simulink model "app_Main1msMgr"  (R2019b)
settings: Solver=FixedStepDiscrete  StartTime=0.0  StopTime=inf  FixedStep=0.001  RelTol=1e-3  EnableMultiTasking=on
PreLoadFcn:
  | try
  |    tapas_types('load');
  | catch
  |   disp('TAPAS WARNING: Tapas Types could not be loaded ...');
  | end
  | 
  | try
  |   app_types('load');
  | catch
  |   currdir =pwd;
  |   try
  |     cd('..\app_types\');
  |     app_types('load');
  |     cd(currdir);
  |   catch
  |     try
  |        cd('..\..\app_types\');
  |        app_types('load');
  |        cd(currdir);
  |     catch
  |        cd(currdir);
  |        disp('TAPAS WARNING: Application Types could not be loaded ...');
  |     end
  |   end
  |   try
  |       clear currdir;
  |   catch
  |      %Do nothing
  |   end
  | end
settings Model: Creator=kmansour  LastModifiedBy=depl_
settings DataIOCC: LimitDataPoints=on  SaveFormat=Array  ReturnWorkspaceOutputs=off
settings OptimizationCC: LifeSpan=1  EfficientTunableParamExpr=on
settings DebuggingCC: AllowSymbolicDim=off  SFUnexpectedBacktrackingDiag=warning  SFNoUnconditionalDefaultTransitionDiag=warning  SFExecutionAtInitializationDiag=none  ArithmeticOperatorsInVariantConditions=warning
settings HardwareCC: ProdBitPerPointer=32  ProdBitPerSizeT=32  ProdBitPerPtrDiffT=32  ProdLargestAtomicInteger=Long  ProdLargestAtomicFloat=Double  ProdEndianess=BigEndian  ProdWordSize=32  ProdHWDeviceType=Texas Instruments->TMS570 Cortex-R4
settings ModelReferenceCC: ModelReferenceNumInstancesAllowed=Single  PropagateSignalLabelsOutOfModel=off
settings SFSimCC: SimUseLocalCustomCode=off  MATLABDynamicMemAlloc=off  CustomCodeUndefinedFunction=UseInterfaceOnly
settings RTWCC: SystemTargetFile=ert.tlc  GenCodeOnly=on  TemplateMakefile=ert_default_tmf  GenerateReport=on  RTWUseLocalCustomCode=off  IncludeHyperlinkInReport=on  LaunchReport=on  GenerateTraceInfo=on  GenerateTraceReport=on  GenerateTraceReportSl=on  GenerateTraceReportSf=on  GenerateTraceReportEml=on
settings CodeAppCC: IgnoreCustomStorageClasses=off  MaxIdLength=63  StateflowObjectComments=on
settings ERTTargetCC: MultiwordLength=2048  GenerateSampleERTMain=on  GenerateASAP2=on  RTWCAPISignals=on  RTWCAPIParams=on  RTWCAPIStates=on  RTWCAPIRootIO=on  ERTSrcFileBannerTemplate=deMCD_code_template.cgt  ERTHdrFileBannerTemplate=deMCD_code_template.cgt  ERTDataSrcFileTemplate=deMCD_code_template.cgt  ERTDataHdrFileTemplate=deMCD_code_template.cgt  ERTCustomFileTemplate=example_file_process.tlc  ConvertIfToSwitch=off  SuppressUnreachableDefaultCases=off
settings ConfigComp: CovMetricSettings=dw  CovHtmlReporting=on  CovSaveCumulativeToWorkspaceVar=on  CovSaveSingleToWorkspaceVar=on  CovExternalEMLEnable=off

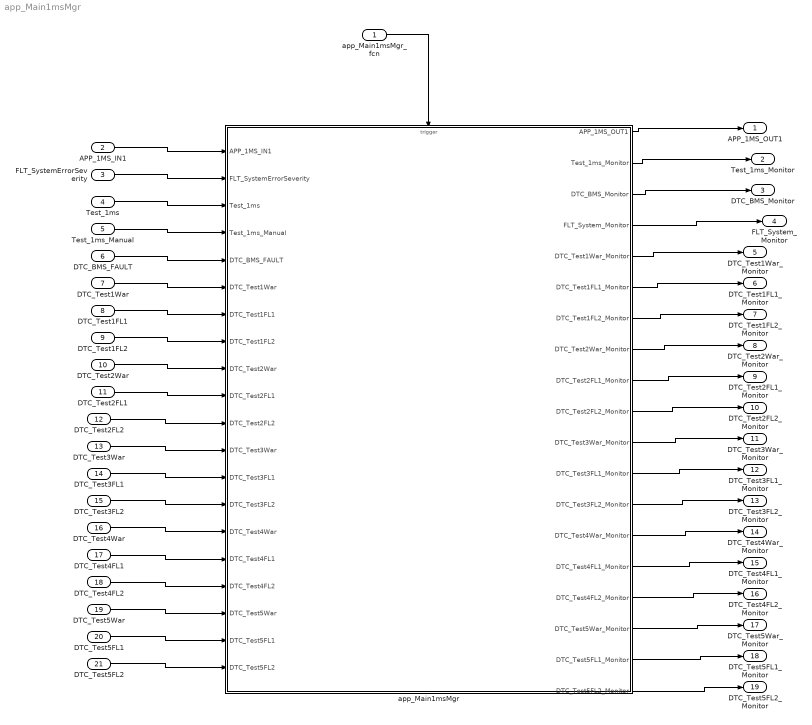
== system app_Main1msMgr ==
  app_Main1msMgr_fcn : Inport  SampleTime=1e-3  OutputFunctionCall=on
  APP_1MS_IN1 : Inport  Port=2
  FLT_SystemErrorSeverity : Inport  Port=3
  Test_1ms : Inport  Port=4
  Test_1ms_Manual : Inport  Port=5
  DTC_BMS_FAULT : Inport  Port=6
  DTC_Test1War : Inport  Port=7
  DTC_Test1FL1 : Inport  Port=8
  DTC_Test1FL2 : Inport  Port=9
  DTC_Test2War : Inport  Port=10
  DTC_Test2FL1 : Inport  Port=11
  DTC_Test2FL2 : Inport  Port=12
  DTC_Test3War : Inport  Port=13
  DTC_Test3FL1 : Inport  Port=14
  DTC_Test3FL2 : Inport  Port=15
  DTC_Test4War : Inport  Port=16
  DTC_Test4FL1 : Inport  Port=17
  DTC_Test4FL2 : Inport  Port=18
  DTC_Test5War : Inport  Port=19
  DTC_Test5FL1 : Inport  Port=20
  DTC_Test5FL2 : Inport  Port=21
  app_Main1msMgr : Subsystem
      mask Display: image(('Devise Logo.JPG'),'center');
  APP_1MS_OUT1 : Outport
  Test_1ms_Monitor : Outport  Port=2
  DTC_BMS_Monitor : Outport  Port=3
  FLT_System_Monitor : Outport  Port=4
  DTC_Test1War_Monitor : Outport  Port=5
  DTC_Test1FL1_Monitor : Outport  Port=6
  DTC_Test1FL2_Monitor : Outport  Port=7
  DTC_Test2War_Monitor : Outport  Port=8
  DTC_Test2FL1_Monitor : Outport  Port=9
  DTC_Test2FL2_Monitor : Outport  Port=10
  DTC_Test3War_Monitor : Outport  Port=11
  DTC_Test3FL1_Monitor : Outport  Port=12
  DTC_Test3FL2_Monitor : Outport  Port=13
  DTC_Test4War_Monitor : Outport  Port=14
  DTC_Test4FL1_Monitor : Outport  Port=15
  DTC_Test4FL2_Monitor : Outport  Port=16
  DTC_Test5War_Monitor : Outport  Port=17
  DTC_Test5FL1_Monitor : Outport  Port=18
  DTC_Test5FL2_Monitor : Outport  Port=19
  wires:
  app_Main1msMgr_fcn/1 -> app_Main1msMgr/Trigger
  APP_1MS_IN1/1 -> app_Main1msMgr/1(APP_1MS_IN1)
  app_Main1msMgr/1(APP_1MS_OUT1) -> APP_1MS_OUT1/1
  FLT_SystemErrorSeverity/1 -> app_Main1msMgr/2(FLT_SystemErrorSeverity)
  Test_1ms/1 -> app_Main1msMgr/3(Test_1ms)
  app_Main1msMgr/2(Test_1ms_Monitor) -> Test_1ms_Monitor/1
  Test_1ms_Manual/1 -> app_Main1msMgr/4(Test_1ms_Manual)
  app_Main1msMgr/3(DTC_BMS_Monitor) -> DTC_BMS_Monitor/1
  app_Main1msMgr/4(FLT_System_Monitor) -> FLT_System_Monitor/1
  DTC_BMS_FAULT/1 -> app_Main1msMgr/5(DTC_BMS_FAULT)
  DTC_Test1War/1 -> app_Main1msMgr/6(DTC_Test1War)
  DTC_Test1FL1/1 -> app_Main1msMgr/7(DTC_Test1FL1)
  DTC_Test1FL2/1 -> app_Main1msMgr/8(DTC_Test1FL2)
  DTC_Test2War/1 -> app_Main1msMgr/9(DTC_Test2War)
  DTC_Test2FL1/1 -> app_Main1msMgr/10(DTC_Test2FL1)
  DTC_Test2FL2/1 -> app_Main1msMgr/11(DTC_Test2FL2)
  DTC_Test3War/1 -> app_Main1msMgr/12(DTC_Test3War)
  DTC_Test3FL1/1 -> app_Main1msMgr/13(DTC_Test3FL1)
  DTC_Test3FL2/1 -> app_Main1msMgr/14(DTC_Test3FL2)
  DTC_Test4War/1 -> app_Main1msMgr/15(DTC_Test4War)
  DTC_Test4FL1/1 -> app_Main1msMgr/16(DTC_Test4FL1)
  DTC_Test4FL2/1 -> app_Main1msMgr/17(DTC_Test4FL2)
  DTC_Test5War/1 -> app_Main1msMgr/18(DTC_Test5War)
  DTC_Test5FL1/1 -> app_Main1msMgr/19(DTC_Test5FL1)
  DTC_Test5FL2/1 -> app_Main1msMgr/20(DTC_Test5FL2)
  app_Main1msMgr/5(DTC_Test1War_Monitor) -> DTC_Test1War_Monitor/1
  app_Main1msMgr/6(DTC_Test1FL1_Monitor) -> DTC_Test1FL1_Monitor/1
  app_Main1msMgr/7(DTC_Test1FL2_Monitor) -> DTC_Test1FL2_Monitor/1
  app_Main1msMgr/8(DTC_Test2War_Monitor) -> DTC_Test2War_Monitor/1
  app_Main1msMgr/9(DTC_Test2FL1_Monitor) -> DTC_Test2FL1_Monitor/1
  app_Main1msMgr/10(DTC_Test2FL2_Monitor) -> DTC_Test2FL2_Monitor/1
  app_Main1msMgr/11(DTC_Test3War_Monitor) -> DTC_Test3War_Monitor/1
  app_Main1msMgr/12(DTC_Test3FL1_Monitor) -> DTC_Test3FL1_Monitor/1
  app_Main1msMgr/13(DTC_Test3FL2_Monitor) -> DTC_Test3FL2_Monitor/1
  app_Main1msMgr/14(DTC_Test4War_Monitor) -> DTC_Test4War_Monitor/1
  app_Main1msMgr/15(DTC_Test4FL1_Monitor) -> DTC_Test4FL1_Monitor/1
  app_Main1msMgr/16(DTC_Test4FL2_Monitor) -> DTC_Test4FL2_Monitor/1
  app_Main1msMgr/17(DTC_Test5War_Monitor) -> DTC_Test5War_Monitor/1
  app_Main1msMgr/18(DTC_Test5FL1_Monitor) -> DTC_Test5FL1_Monitor/1
  app_Main1msMgr/19(DTC_Test5FL2_Monitor) -> DTC_Test5FL2_Monitor/1

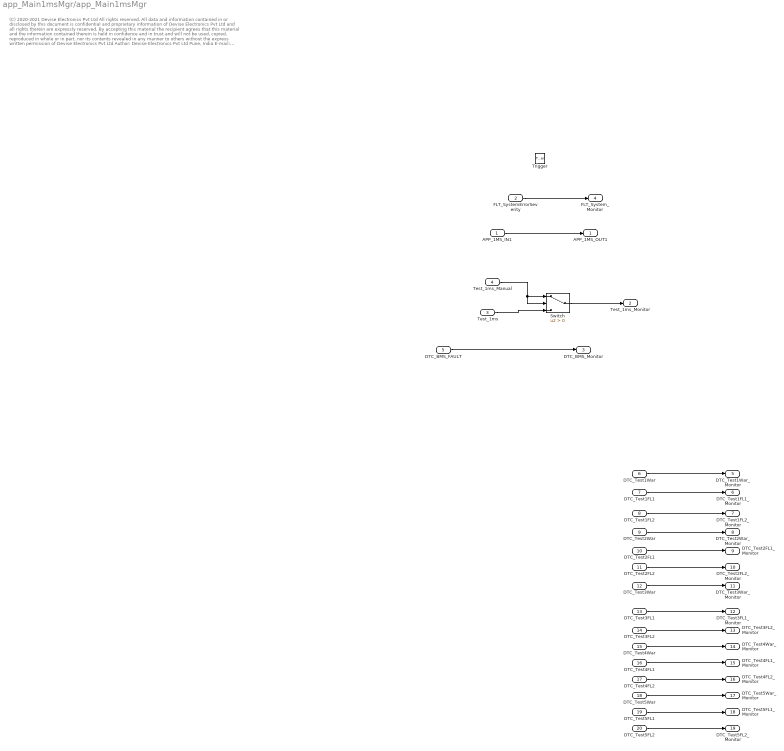
== system app_Main1msMgr/app_Main1msMgr ==
  note: (C) 2020-2021 Devise Electronics Pvt Ltd
      | All rights reserved.
      |
      | All data and information contained in or disclosed by this document is confidential and proprietary information of Devise Electronics Pvt Ltd and all rights therein are expressly reserved. By accepting this material the recipient agrees that this material and the information contained therein is held in confidence and in trust and will not be used, copied, reproduced in whole or in part, nor its contents revealed in any manner to others without the express written permission of Devise Electronics Pvt Ltd
      |
      | Author:
      |
      | Devise Electronics Pvt Ltd
      | Pune,
      | India
      | E-mail: Shekhar.malani@deviseelectronics.com
  APP_1MS_IN1 : Inport
  FLT_SystemErrorSeverity : Inport  Port=2
  Test_1ms : Inport  Port=3
  Test_1ms_Manual : Inport  Port=4
  DTC_BMS_FAULT : Inport  Port=5
  DTC_Test1War : Inport  Port=6
  DTC_Test1FL1 : Inport  Port=7
  DTC_Test1FL2 : Inport  Port=8
  DTC_Test2War : Inport  Port=9
  DTC_Test2FL1 : Inport  Port=10
  DTC_Test2FL2 : Inport  Port=11
  DTC_Test3War : Inport  Port=12
  DTC_Test3FL1 : Inport  Port=13
  DTC_Test3FL2 : Inport  Port=14
  DTC_Test4War : Inport  Port=15
  DTC_Test4FL1 : Inport  Port=16
  DTC_Test4FL2 : Inport  Port=17
  DTC_Test5War : Inport  Port=18
  DTC_Test5FL1 : Inport  Port=19
  DTC_Test5FL2 : Inport  Port=20
  Trigger : TriggerPort  TriggerType=function-call  VariantControl=Variant  SampleTimeType=periodic  SampleTime=-1  PortDimensions=1
  Switch : Switch  Criteria=u2 > Threshold
  APP_1MS_OUT1 : Outport
  Test_1ms_Monitor : Outport  Port=2
  DTC_BMS_Monitor : Outport  Port=3
  FLT_System_Monitor : Outport  Port=4
  DTC_Test1War_Monitor : Outport  Port=5
  DTC_Test1FL1_Monitor : Outport  Port=6
  DTC_Test1FL2_Monitor : Outport  Port=7
  DTC_Test2War_Monitor : Outport  Port=8
  DTC_Test2FL1_Monitor : Outport  Port=9
  DTC_Test2FL2_Monitor : Outport  Port=10
  DTC_Test3War_Monitor : Outport  Port=11
  DTC_Test3FL1_Monitor : Outport  Port=12
  DTC_Test3FL2_Monitor : Outport  Port=13
  DTC_Test4War_Monitor : Outport  Port=14
  DTC_Test4FL1_Monitor : Outport  Port=15
  DTC_Test4FL2_Monitor : Outport  Port=16
  DTC_Test5War_Monitor : Outport  Port=17
  DTC_Test5FL1_Monitor : Outport  Port=18
  DTC_Test5FL2_Monitor : Outport  Port=19
  wires:
  APP_1MS_IN1/1 -> APP_1MS_OUT1/1
  FLT_SystemErrorSeverity/1 -> FLT_System_Monitor/1
  Test_1ms/1 -> Switch/3
  Switch/1 -> Test_1ms_Monitor/1
  Test_1ms_Manual/1 -> Switch/2, Switch/1
  DTC_BMS_FAULT/1 -> DTC_BMS_Monitor/1
  DTC_Test2FL2/1 -> DTC_Test2FL2_Monitor/1
  DTC_Test3War/1 -> DTC_Test3War_Monitor/1
  DTC_Test5FL2/1 -> DTC_Test5FL2_Monitor/1
  DTC_Test5FL1/1 -> DTC_Test5FL1_Monitor/1
  DTC_Test5War/1 -> DTC_Test5War_Monitor/1
  DTC_Test4FL2/1 -> DTC_Test4FL2_Monitor/1
  DTC_Test4FL1/1 -> DTC_Test4FL1_Monitor/1
  DTC_Test4War/1 -> DTC_Test4War_Monitor/1
  DTC_Test3FL2/1 -> DTC_Test3FL2_Monitor/1
  DTC_Test3FL1/1 -> DTC_Test3FL1_Monitor/1
  DTC_Test2FL1/1 -> DTC_Test2FL1_Monitor/1
  DTC_Test2War/1 -> DTC_Test2War_Monitor/1
  DTC_Test1FL2/1 -> DTC_Test1FL2_Monitor/1
  DTC_Test1FL1/1 -> DTC_Test1FL1_Monitor/1
  DTC_Test1War/1 -> DTC_Test1War_Monitor/1
